simulink model "PE_main"  (R2025b)
settings: Solver=ode4  StartTime=0.0  StopTime=600  FixedStep=0.001  RelTol=1e-3
libraries: simulink x1
settings Model: Creator=manikantagonugondla  LastModifiedBy=manikantagonugondla

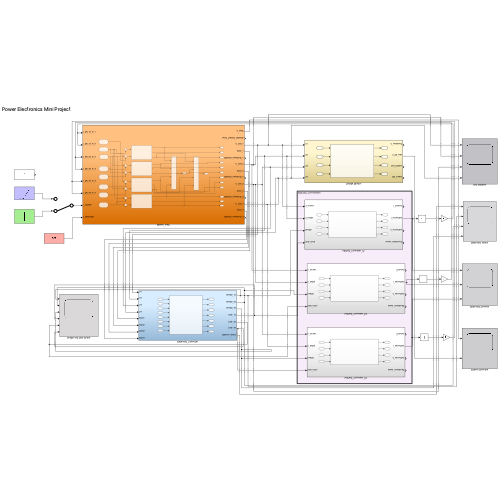
[thumbnail: Simulink's stored preview of the top-level diagram]
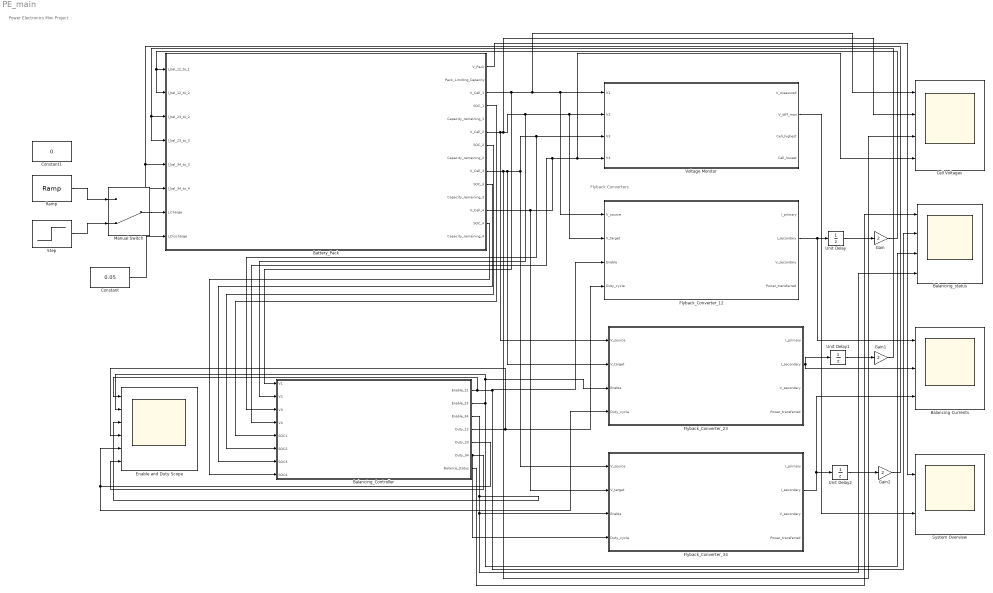
== system PE_main ==
  note: Power Electronics Mini Project
  note: Flyback Converters
  Balancing Currents : Scope  NumInputPorts=3
      settings: ActiveDisplayYMinimum=-7.6961589180783845  ActiveDisplayYMaximum=7.5868246502245036  DataLoggingVariableName=ScopeData2
  Balancing_Controller : Subsystem
  Balancing_status : Scope  NumInputPorts=4
      settings: ActiveDisplayYMinimum=1.1215595122943847  ActiveDisplayYMaximum=2.0976044986339573
  Battery_Pack : Subsystem
  Cell Voltages : Scope  NumInputPorts=4
      settings: ActiveDisplayYMinimum=2.624907670031094  ActiveDisplayYMaximum=4.321195310518152
  Constant : Constant  Value=0.05
  Constant1 : Constant  Value=0
  Enable and Duty Scope : Scope  NumInputPorts=6
      settings: ActiveDisplayYMinimum=-0.12499999999999997  ActiveDisplayYMaximum=1.125  DataLoggingVariableName=ScopeData4
  Flyback_Converter_12 : Subsystem
  Flyback_Converter_23 : Subsystem
  Flyback_Converter_34 : Subsystem
  Gain : Gain  Gain=2
  Gain1 : Gain  Gain=2
  Gain2 : Gain  Gain=2
  Manual Switch : ManualSwitch  CurrentSetting=0
  Ramp : simulink/Sources/Ramp  slope=0.01  start=100  InitialOutput=0
  Step : Step  Time=200  After=0.5  SampleTime=0
  System Overview : Scope  NumInputPorts=2
      settings: ActiveDisplayYMinimum=13.339480983921661  ActiveDisplayYMaximum=13.76875860674742  DataLoggingVariableName=ScopeData3
  Unit Delay : UnitDelay  SampleTime=-1  HasFrameUpgradeWarning=on
  Unit Delay1 : UnitDelay  SampleTime=-1  HasFrameUpgradeWarning=on
  Unit Delay2 : UnitDelay  SampleTime=-1  HasFrameUpgradeWarning=on
  Voltage Monitor : Subsystem
  wires:
  Battery_Pack/9(V_Cell_3) -> Cell Voltages/3, Flyback_Converter_23/2(V_target), Balancing_Controller/3(V3), Voltage Monitor/3(V3), Flyback_Converter_34/1(V_source)
  Battery_Pack/12(V_Cell_4) -> Flyback_Converter_34/2(V_target), Balancing_Controller/4(V4), Cell Voltages/4, Voltage Monitor/4(V4)
  Battery_Pack/4(SOC_1) -> Balancing_Controller/5(SOC1)
  Battery_Pack/7(SOC_2) -> Balancing_Controller/6(SOC2)
  Battery_Pack/10(SOC_3) -> Balancing_Controller/7(SOC3)
  Battery_Pack/13(SOC_4) -> Balancing_Controller/8(SOC4)
  Balancing_Controller/2(Enable_23) -> Enable and Duty Scope/2, Flyback_Converter_23/3(Enable), Balancing_status/3
  Balancing_Controller/3(Enable_34) -> Balancing_status/4, Flyback_Converter_34/3(Enable), Enable and Duty Scope/3
  Balancing_Controller/5(Duty_23) -> Enable and Duty Scope/5, Flyback_Converter_23/4(Duty_cycle)
  Balancing_Controller/6(Duty_34) -> Enable and Duty Scope/6, Flyback_Converter_34/4(Duty_cycle)
  Balancing_Controller/7(Balance_status) -> Balancing_status/1
  Flyback_Converter_12/2(I_secondary) -> Unit Delay/1, Balancing Currents/1
  Flyback_Converter_23/2(I_secondary) -> Unit Delay1/1, Balancing Currents/2
  Flyback_Converter_34/2(I_secondary) -> Balancing Currents/3, Unit Delay2/1
  Battery_Pack/1(V_Pack) -> System Overview/1
  Voltage Monitor/2(V_diff_max) -> System Overview/2
  Constant/1 -> Battery_Pack/8(I_Discharge)
  Gain/1 -> Battery_Pack/2(I_bal_12_to_2), Battery_Pack/1(I_bal_12_to_1)
  Gain2/1 -> Battery_Pack/6(I_bal_34_to_4), Battery_Pack/5(I_bal_34_to_3)
  Unit Delay/1 -> Gain/1
  Unit Delay1/1 -> Gain1/1
  Unit Delay2/1 -> Gain2/1
  Gain1/1 -> Battery_Pack/4(I_bal_23_to_3), Battery_Pack/3(I_bal_23_to_2)
  Battery_Pack/6(V_Cell_2) -> Flyback_Converter_23/1(V_source), Cell Voltages/2, Balancing_Controller/2(V2), Flyback_Converter_12/2(V_target), Voltage Monitor/2(V2)
  Battery_Pack/3(V_Cell_1) -> Balancing_Controller/1(V1), Cell Voltages/1, Flyback_Converter_12/1(V_source), Voltage Monitor/1(V1)
  Balancing_Controller/1(Enable_12) -> Enable and Duty Scope/1, Flyback_Converter_12/3(Enable), Balancing_status/2
  Balancing_Controller/4(Duty_12) -> Enable and Duty Scope/4, Flyback_Converter_12/4(Duty_cycle)
  Ramp/1 -> Manual Switch/1
  Step/1 -> Manual Switch/2
  Manual Switch/1 -> Battery_Pack/7(I_Charge)

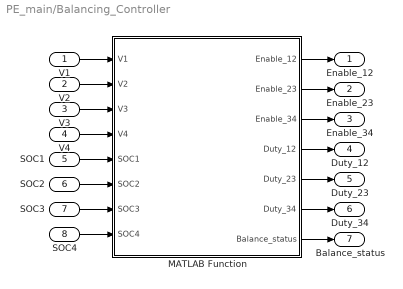
== system PE_main/Balancing_Controller ==
  V1 : Inport
  V2 : Inport  Port=2
  V3 : Inport  Port=3
  V4 : Inport  Port=4
  SOC1 : Inport  Port=5
  SOC2 : Inport  Port=6
  SOC3 : Inport  Port=7
  SOC4 : Inport  Port=8
  MATLAB Function : MATLAB Function  TreatAsAtomicUnit=on
  Enable_12 : Outport
  Enable_23 : Outport  Port=2
  Enable_34 : Outport  Port=3
  Duty_12 : Outport  Port=4
  Duty_23 : Outport  Port=5
  Duty_34 : Outport  Port=6
  Balance_status : Outport  Port=7
  wires:
  V1/1 -> MATLAB Function/1(V1)
  MATLAB Function/1(Enable_12) -> Enable_12/1
  V2/1 -> MATLAB Function/2(V2)
  V3/1 -> MATLAB Function/3(V3)
  V4/1 -> MATLAB Function/4(V4)
  SOC1/1 -> MATLAB Function/5(SOC1)
  SOC2/1 -> MATLAB Function/6(SOC2)
  SOC3/1 -> MATLAB Function/7(SOC3)
  SOC4/1 -> MATLAB Function/8(SOC4)
  MATLAB Function/2(Enable_23) -> Enable_23/1
  MATLAB Function/3(Enable_34) -> Enable_34/1
  MATLAB Function/4(Duty_12) -> Duty_12/1
  MATLAB Function/5(Duty_23) -> Duty_23/1
  MATLAB Function/6(Duty_34) -> Duty_34/1
  MATLAB Function/7(Balance_status) -> Balance_status/1

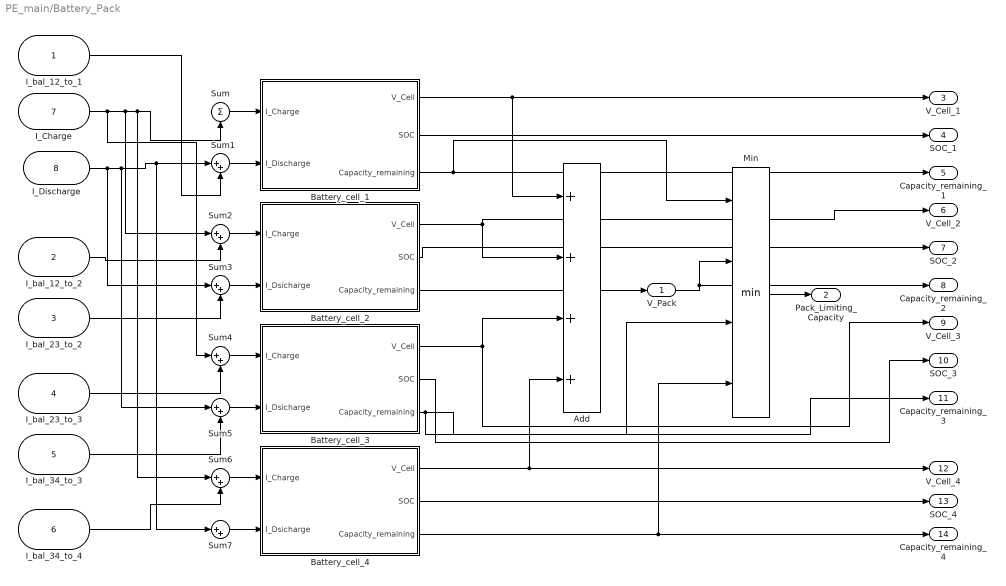
== system PE_main/Battery_Pack ==
  I_bal_12_to_1 : Inport
  I_bal_12_to_2 : Inport  Port=2
  I_bal_23_to_2 : Inport  Port=3
  I_bal_23_to_3 : Inport  Port=4
  I_bal_34_to_3 : Inport  Port=5
  I_bal_34_to_4 : Inport  Port=6
  I_Charge : Inport  Port=7
  I_Discharge : Inport  Port=8
  Add : Sum  Inputs=++++
  Battery_cell_1 : Subsystem
  Battery_cell_2 : Subsystem
  Battery_cell_3 : Subsystem
  Battery_cell_4 : Subsystem
  Min : MinMax  Inputs=4
  Sum : Sum  Inputs=|+
  Sum{1..7} (7 alike) : Sum  Inputs=|++
  V_Pack : Outport
  Pack_Limiting_Capacity : Outport  Port=2
  V_Cell_1 : Outport  Port=3
  SOC_1 : Outport  Port=4
  Capacity_remaining_1 : Outport  Port=5
  V_Cell_2 : Outport  Port=6
  SOC_2 : Outport  Port=7
  Capacity_remaining_2 : Outport  Port=8
  V_Cell_3 : Outport  Port=9
  SOC_3 : Outport  Port=10
  Capacity_remaining_3 : Outport  Port=11
  V_Cell_4 : Outport  Port=12
  SOC_4 : Outport  Port=13
  Capacity_remaining_4 : Outport  Port=14
  wires:
  Battery_cell_1/1(V_Cell) -> V_Cell_1/1, Add/1
  Battery_cell_2/1(V_Cell) -> Add/2, V_Cell_2/1
  Battery_cell_3/1(V_Cell) -> Add/3, V_Cell_3/1
  Battery_cell_4/1(V_Cell) -> V_Cell_4/1, Add/4
  Add/1 -> V_Pack/1
  Battery_cell_1/3(Capacity_remaining) -> Min/1, Capacity_remaining_1/1
  Battery_cell_2/3(Capacity_remaining) -> Min/2, Capacity_remaining_2/1
  Battery_cell_3/3(Capacity_remaining) -> Capacity_remaining_3/1, Min/3
  Battery_cell_4/3(Capacity_remaining) -> Capacity_remaining_4/1, Min/4
  Min/1 -> Pack_Limiting_Capacity/1
  Battery_cell_1/2(SOC) -> SOC_1/1
  Battery_cell_2/2(SOC) -> SOC_2/1
  Battery_cell_3/2(SOC) -> SOC_3/1
  Battery_cell_4/2(SOC) -> SOC_4/1
  I_Charge/1 -> Sum4/1, Sum2/1, Sum6/1, Sum/1
  Sum/1 -> Battery_cell_1/1(I_Charge)
  I_bal_12_to_1/1 -> Sum1/2
  I_Discharge/1 -> Sum5/1, Sum7/1, Sum1/1, Sum3/1
  Sum1/1 -> Battery_cell_1/2(I_Discharge)
  Sum2/1 -> Battery_cell_2/1(I_Charge)
  I_bal_12_to_2/1 -> Sum2/2
  I_bal_23_to_2/1 -> Sum3/2
  Sum3/1 -> Battery_cell_2/2(I_Dsicharge)
  I_bal_23_to_3/1 -> Sum4/2
  I_bal_34_to_3/1 -> Sum5/2
  I_bal_34_to_4/1 -> Sum6/2
  Sum4/1 -> Battery_cell_3/1(I_Charge)
  Sum5/1 -> Battery_cell_3/2(I_Dsicharge)
  Sum6/1 -> Battery_cell_4/1(I_Charge)
  Sum7/1 -> Battery_cell_4/2(I_Dsicharge)

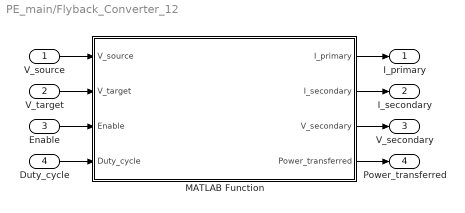
== system PE_main/Flyback_Converter_12 ==
  V_source : Inport
  V_target : Inport  Port=2
  Enable : Inport  Port=3
  Duty_cycle : Inport  Port=4
  MATLAB Function : MATLAB Function  TreatAsAtomicUnit=on
  I_primary : Outport
  I_secondary : Outport  Port=2
  V_secondary : Outport  Port=3
  Power_transferred : Outport  Port=4
  wires:
  V_source/1 -> MATLAB Function/1(V_source)
  MATLAB Function/1(I_primary) -> I_primary/1
  Enable/1 -> MATLAB Function/3(Enable)
  Duty_cycle/1 -> MATLAB Function/4(Duty_cycle)
  MATLAB Function/3(V_secondary) -> V_secondary/1
  MATLAB Function/2(I_secondary) -> I_secondary/1
  MATLAB Function/4(Power_transferred) -> Power_transferred/1
  V_target/1 -> MATLAB Function/2(V_target)

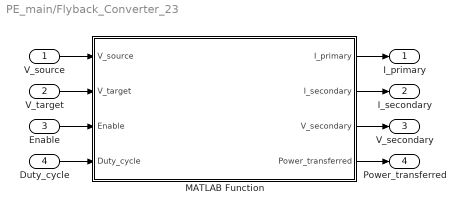
== system PE_main/Flyback_Converter_23 ==
  V_source : Inport
  V_target : Inport  Port=2
  Enable : Inport  Port=3
  Duty_cycle : Inport  Port=4
  MATLAB Function : MATLAB Function  TreatAsAtomicUnit=on
  I_primary : Outport
  I_secondary : Outport  Port=2
  V_secondary : Outport  Port=3
  Power_transferred : Outport  Port=4
  wires:
  V_source/1 -> MATLAB Function/1(V_source)
  MATLAB Function/1(I_primary) -> I_primary/1
  Enable/1 -> MATLAB Function/3(Enable)
  Duty_cycle/1 -> MATLAB Function/4(Duty_cycle)
  MATLAB Function/3(V_secondary) -> V_secondary/1
  MATLAB Function/2(I_secondary) -> I_secondary/1
  MATLAB Function/4(Power_transferred) -> Power_transferred/1
  V_target/1 -> MATLAB Function/2(V_target)

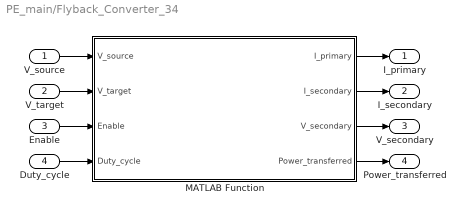
== system PE_main/Flyback_Converter_34 ==
  V_source : Inport
  V_target : Inport  Port=2
  Enable : Inport  Port=3
  Duty_cycle : Inport  Port=4
  MATLAB Function : MATLAB Function  TreatAsAtomicUnit=on
  I_primary : Outport
  I_secondary : Outport  Port=2
  V_secondary : Outport  Port=3
  Power_transferred : Outport  Port=4
  wires:
  V_source/1 -> MATLAB Function/1(V_source)
  MATLAB Function/1(I_primary) -> I_primary/1
  Enable/1 -> MATLAB Function/3(Enable)
  Duty_cycle/1 -> MATLAB Function/4(Duty_cycle)
  MATLAB Function/3(V_secondary) -> V_secondary/1
  MATLAB Function/2(I_secondary) -> I_secondary/1
  MATLAB Function/4(Power_transferred) -> Power_transferred/1
  V_target/1 -> MATLAB Function/2(V_target)

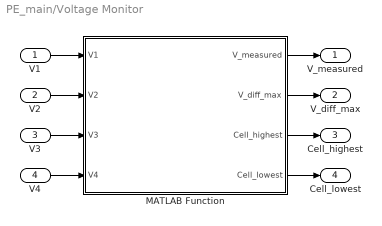
== system PE_main/Voltage Monitor ==
  V1 : Inport
  V2 : Inport  Port=2
  V3 : Inport  Port=3
  V4 : Inport  Port=4
  MATLAB Function : MATLAB Function  TreatAsAtomicUnit=on
  V_measured : Outport
  V_diff_max : Outport  Port=2
  Cell_highest : Outport  Port=3
  Cell_lowest : Outport  Port=4
  wires:
  V1/1 -> MATLAB Function/1(V1)
  V2/1 -> MATLAB Function/2(V2)
  V3/1 -> MATLAB Function/3(V3)
  V4/1 -> MATLAB Function/4(V4)
  MATLAB Function/2(V_diff_max) -> V_diff_max/1
  MATLAB Function/3(Cell_highest) -> Cell_highest/1
  MATLAB Function/1(V_measured) -> V_measured/1
  MATLAB Function/4(Cell_lowest) -> Cell_lowest/1

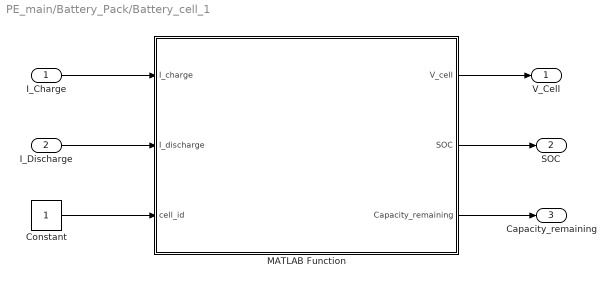
== system PE_main/Battery_Pack/Battery_cell_1 ==
  I_Charge : Inport
  I_Discharge : Inport  Port=2
  Constant : Constant
  MATLAB Function : MATLAB Function  TreatAsAtomicUnit=on
  V_Cell : Outport
  SOC : Outport  Port=2
  Capacity_remaining : Outport  Port=3
  wires:
  I_Discharge/1 -> MATLAB Function/2(I_discharge)
  I_Charge/1 -> MATLAB Function/1(I_charge)
  MATLAB Function/1(V_cell) -> V_Cell/1
  MATLAB Function/2(SOC) -> SOC/1
  MATLAB Function/3(Capacity_remaining) -> Capacity_remaining/1
  Constant/1 -> MATLAB Function/3(cell_id)

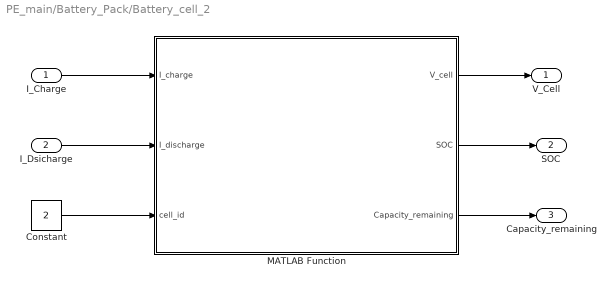
== system PE_main/Battery_Pack/Battery_cell_2 ==
  I_Charge : Inport
  I_Dsicharge : Inport  Port=2
  Constant : Constant  Value=2
  MATLAB Function : MATLAB Function  TreatAsAtomicUnit=on
  V_Cell : Outport
  SOC : Outport  Port=2
  Capacity_remaining : Outport  Port=3
  wires:
  I_Dsicharge/1 -> MATLAB Function/2(I_discharge)
  I_Charge/1 -> MATLAB Function/1(I_charge)
  MATLAB Function/1(V_cell) -> V_Cell/1
  MATLAB Function/2(SOC) -> SOC/1
  MATLAB Function/3(Capacity_remaining) -> Capacity_remaining/1
  Constant/1 -> MATLAB Function/3(cell_id)

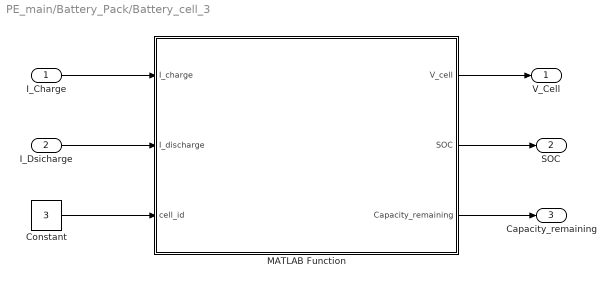
== system PE_main/Battery_Pack/Battery_cell_3 ==
  I_Charge : Inport
  I_Dsicharge : Inport  Port=2
  Constant : Constant  Value=3
  MATLAB Function : MATLAB Function  TreatAsAtomicUnit=on
  V_Cell : Outport
  SOC : Outport  Port=2
  Capacity_remaining : Outport  Port=3
  wires:
  I_Dsicharge/1 -> MATLAB Function/2(I_discharge)
  I_Charge/1 -> MATLAB Function/1(I_charge)
  MATLAB Function/1(V_cell) -> V_Cell/1
  MATLAB Function/2(SOC) -> SOC/1
  MATLAB Function/3(Capacity_remaining) -> Capacity_remaining/1
  Constant/1 -> MATLAB Function/3(cell_id)

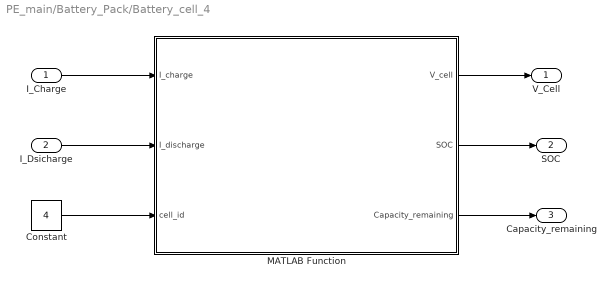
== system PE_main/Battery_Pack/Battery_cell_4 ==
  I_Charge : Inport
  I_Dsicharge : Inport  Port=2
  Constant : Constant  Value=4
  MATLAB Function : MATLAB Function  TreatAsAtomicUnit=on
  V_Cell : Outport
  SOC : Outport  Port=2
  Capacity_remaining : Outport  Port=3
  wires:
  I_Dsicharge/1 -> MATLAB Function/2(I_discharge)
  I_Charge/1 -> MATLAB Function/1(I_charge)
  MATLAB Function/1(V_cell) -> V_Cell/1
  MATLAB Function/2(SOC) -> SOC/1
  MATLAB Function/3(Capacity_remaining) -> Capacity_remaining/1
  Constant/1 -> MATLAB Function/3(cell_id)

== matlab function PE_main/Flyback_Converter_23/MATLAB Function ==
  data: V_source input; I_primary output; V_target input; Enable input; Duty_cycle input; I_secondary output; V_secondary output; Power_transferred output
function [I_primary, I_secondary, V_secondary, Power_transferred] = flyback_converter(V_source, V_target, Enable, Duty_cycle)
% Bidirectional Flyback Converter Model
% Automatically determines energy transfer direction based on voltage difference
% Energy flows from higher voltage cell to lower voltage cell

% Converter Parameters
L_primary = 100e-6;           % Primary inductance (100 µH)
N_ratio = 1.0;                % Turns ratio (1:1)
R_primary = 0.1;              % Primary winding resistance (Ohm)
R_secondary = 0.1;            % Secondary winding resistance (Ohm)
f_switching = 50e3;           % Switching frequency (50 kHz)
V_mosfet_drop = 0.1;          % MOSFET voltage drop (V)
V_diode_drop = 0.3;           % Diode voltage drop (V)
efficiency = 0.9;             % Energy transfer efficiency (90%)

% Persistent state variables
persistent I_L_state t_state;
if isempty(I_L_state)
    I_L_state = 0.0;
    t_state = 0.0;
end

% Time step and switching period
dt = 1e-5;                    % Fixed time step (10 µs)
t_state = t_state + dt;
T_switching = 1/f_switching;
t_normalized = mod(t_state, T_switching) / T_switching;

% Initialize outputs
I_primary = 0.0;
I_secondary = 0.0;
V_secondary = 0.0;
Power_transferred = 0.0;

% Determine energy transfer direction
V_diff = V_source - V_target;
voltage_threshold = 0.01;     % Minimum 10 mV difference to operate

% Check if converter should be active
converter_active = (Enable > 0.5) && (abs(V_diff) > voltage_threshold) && (Duty_cycle > 0.01);

if ~converter_active
    % Converter disabled - reset inductor current
    I_L_state = 0;
    return;
end

% Determine which cell is higher voltage (energy source)
if V_diff > 0
    % V_source > V_target: Forward direction
    % Energy flows from source to target
    V_high = V_source;
    V_low = V_target;
    direction = 1;  % Forward
else
    % V_target > V_source: Reverse direction
    % Energy flows from target to source
    V_high = V_target;
    V_low = V_source;
    direction = -1; % Reverse
end

% Generate switching signal
switch_on = (t_normalized < Duty_cycle);

if switch_on
    % ===== ENERGY STORAGE PHASE =====
    % MOSFET ON: Current builds up in primary inductance
    % Energy is stored in the magnetic field
    
    % Voltage across inductor (from high voltage cell)
    V_inductor = V_high - I_L_state * R_primary - V_mosfet_drop;
    
    % Rate of current change: V = L * di/dt
    dI_dt = V_inductor / L_primary;
    
    % Update inductor current
    I_L_state = max(0, I_L_state + dI_dt * dt);
    
    % Current flows through primary during this phase
    if direction > 0
        I_primary = I_L_state;
        I_secondary = 0;
    else
        I_primary = 0;
        I_secondary = -I_L_state; % Negative indicates reverse flow
    end
    
else
    % ===== ENERGY TRANSFER PHASE =====
    % MOSFET OFF: Stored energy transfers to secondary
    % Inductor current flows through secondary winding to low voltage cell
    
    if I_L_state > 0.01  % Only transfer if sufficient current exists
        
        % Calculate secondary current with transformer ratio and efficiency
        I_transferred = I_L_state * N_ratio * efficiency;
        
        % Voltage at secondary side
        V_secondary_actual = V_low + I_transferred * R_secondary + V_diode_drop;
        
        if direction > 0
            % Forward: Energy to target
            I_primary = 0;
            I_secondary = I_transferred;
            V_secondary = V_secondary_actual;
        else
            % Reverse: Energy to source
            I_primary = -I_transferred;
            I_secondary = 0;
            V_secondary = V_secondary_actual;
        end
        
        % Decay inductor current (energy has been transferred)
        % Exponential decay model
        decay_factor = 0.95;  % Faster decay for realistic behavior
        I_L_state = I_L_state * decay_factor;
        
    else
        % Current too low - reset
        I_L_state = 0;
    end
end

% Calculate instantaneous power transfer
if direction > 0
    Power_transferred = abs(I_secondary * V_target);
else
    Power_transferred = abs(I_primary * V_source);
end

end

== matlab function PE_main/Flyback_Converter_34/MATLAB Function ==
  data: V_source input; I_primary output; V_target input; Enable input; Duty_cycle input; I_secondary output; V_secondary output; Power_transferred output
function [I_primary, I_secondary, V_secondary, Power_transferred] = flyback_converter(V_source, V_target, Enable, Duty_cycle)
% Bidirectional Flyback Converter Model
% Automatically determines energy transfer direction based on voltage difference
% Energy flows from higher voltage cell to lower voltage cell

% Converter Parameters
L_primary = 100e-6;           % Primary inductance (100 µH)
N_ratio = 1.0;                % Turns ratio (1:1)
R_primary = 0.1;              % Primary winding resistance (Ohm)
R_secondary = 0.1;            % Secondary winding resistance (Ohm)
f_switching = 50e3;           % Switching frequency (50 kHz)
V_mosfet_drop = 0.1;          % MOSFET voltage drop (V)
V_diode_drop = 0.3;           % Diode voltage drop (V)
efficiency = 0.9;             % Energy transfer efficiency (90%)

% Persistent state variables
persistent I_L_state t_state;
if isempty(I_L_state)
    I_L_state = 0.0;
    t_state = 0.0;
end

% Time step and switching period
dt = 1e-5;                    % Fixed time step (10 µs)
t_state = t_state + dt;
T_switching = 1/f_switching;
t_normalized = mod(t_state, T_switching) / T_switching;

% Initialize outputs
I_primary = 0.0;
I_secondary = 0.0;
V_secondary = 0.0;
Power_transferred = 0.0;

% Determine energy transfer direction
V_diff = V_source - V_target;
voltage_threshold = 0.01;     % Minimum 10 mV difference to operate

% Check if converter should be active
converter_active = (Enable > 0.5) && (abs(V_diff) > voltage_threshold) && (Duty_cycle > 0.01);

if ~converter_active
    % Converter disabled - reset inductor current
    I_L_state = 0;
    return;
end

% Determine which cell is higher voltage (energy source)
if V_diff > 0
    % V_source > V_target: Forward direction
    % Energy flows from source to target
    V_high = V_source;
    V_low = V_target;
    direction = 1;  % Forward
else
    % V_target > V_source: Reverse direction
    % Energy flows from target to source
    V_high = V_target;
    V_low = V_source;
    direction = -1; % Reverse
end

% Generate switching signal
switch_on = (t_normalized < Duty_cycle);

if switch_on
    % ===== ENERGY STORAGE PHASE =====
    % MOSFET ON: Current builds up in primary inductance
    % Energy is stored in the magnetic field
    
    % Voltage across inductor (from high voltage cell)
    V_inductor = V_high - I_L_state * R_primary - V_mosfet_drop;
    
    % Rate of current change: V = L * di/dt
    dI_dt = V_inductor / L_primary;
    
    % Update inductor current
    I_L_state = max(0, I_L_state + dI_dt * dt);
    
    % Current flows through primary during this phase
    if direction > 0
        I_primary = I_L_state;
        I_secondary = 0;
    else
        I_primary = 0;
        I_secondary = -I_L_state; % Negative indicates reverse flow
    end
    
else
    % ===== ENERGY TRANSFER PHASE =====
    % MOSFET OFF: Stored energy transfers to secondary
    % Inductor current flows through secondary winding to low voltage cell
    
    if I_L_state > 0.01  % Only transfer if sufficient current exists
        
        % Calculate secondary current with transformer ratio and efficiency
        I_transferred = I_L_state * N_ratio * efficiency;
        
        % Voltage at secondary side
        V_secondary_actual = V_low + I_transferred * R_secondary + V_diode_drop;
        
        if direction > 0
            % Forward: Energy to target
            I_primary = 0;
            I_secondary = I_transferred;
            V_secondary = V_secondary_actual;
        else
            % Reverse: Energy to source
            I_primary = -I_transferred;
            I_secondary = 0;
            V_secondary = V_secondary_actual;
        end
        
        % Decay inductor current (energy has been transferred)
        % Exponential decay model
        decay_factor = 0.95;  % Faster decay for realistic behavior
        I_L_state = I_L_state * decay_factor;
        
    else
        % Current too low - reset
        I_L_state = 0;
    end
end

% Calculate instantaneous power transfer
if direction > 0
    Power_transferred = abs(I_secondary * V_target);
else
    Power_transferred = abs(I_primary * V_source);
end

end

== matlab function PE_main/Battery_Pack/Battery_cell_1/MATLAB Function ==
  data: I_charge input; V_cell output; I_discharge input; SOC output; Capacity_remaining output; cell_id input
function [V_cell, SOC, Capacity_remaining] = battery_cell_model(I_charge, I_discharge, cell_id)
%#codegen
% Lithium-ion Battery Cell Model
% Models voltage, SOC, and capacity with realistic variations

% Persistent state variables (retain values between function calls)
persistent SOC_state Capacity_Ah_state;

% Initialize persistent variables on first run
if isempty(SOC_state)
    % Set initial SOC based on cell ID to create imbalance
    if cell_id == 1
        SOC_state = 0.65;     % Cell 1: 65% SOC
    elseif cell_id == 2
        SOC_state = 0.70;     % Cell 2: 70% SOC (highest)
    elseif cell_id == 3
        SOC_state = 0.55;     % Cell 3: 55% SOC (lowest)
    else
        SOC_state = 0.60;     % Cell 4: 60% SOC
    end
end

if isempty(Capacity_Ah_state)
    % Cell capacities vary by ±5% (realistic manufacturing variation)
    base_capacity = 2.5;      % 2.5 Ah base capacity
    
    if cell_id == 1
        capacity_factor = 1.02;  % +2% (2.55 Ah)
    elseif cell_id == 2
        capacity_factor = 0.98;  % -2% (2.45 Ah)
    elseif cell_id == 3
        capacity_factor = 1.05;  % +5% (2.625 Ah)
    else
        capacity_factor = 0.97;  % -3% (2.425 Ah)
    end
    
    Capacity_Ah_state = base_capacity * capacity_factor;
end

% ===== BATTERY PARAMETERS =====
V_nominal = 3.7;              % Nominal voltage (V)
V_max = 4.2;                  % Maximum safe voltage (V)
V_min = 2.5;                  % Minimum safe voltage (V)
R_internal_base = 0.05;       % Base internal resistance (Ohm)
alpha = 0.3;                  % Resistance variation coefficient

% Internal resistance varies with SOC (increases as SOC decreases)
R_internal = R_internal_base * (1.0 + alpha * (1.0 - SOC_state));

% ===== NET CURRENT CALCULATION =====
% Positive I_net = charging, Negative I_net = discharging
I_net = I_charge - I_discharge;

% ===== SOC UPDATE =====
% Update SOC using current integration (Coulomb counting)
dt = 0.001;                   % Integration time step (1 ms)
dSOC = (I_net * dt) / (Capacity_Ah_state * 3600.0);  % Convert Ah to As
SOC_state = SOC_state + dSOC;

% Limit SOC to physical bounds [0, 1]
SOC_state = max(min(SOC_state, 1.0), 0.0);

% ===== OPEN CIRCUIT VOLTAGE CALCULATION =====
% Non-linear relationship between SOC and voltage
if SOC_state > 0.95
    % High SOC region (95-100%): voltage increases rapidly
    V_oc = V_max - 0.1 * (1.0 - SOC_state) / 0.05;
elseif SOC_state > 0.1
    % Normal operating region (10-95%): approximately linear
    V_oc = V_min + (V_nominal - V_min) * (SOC_state - 0.1) / 0.85 + 0.3 * SOC_state;
else
    % Low SOC region (0-10%): voltage drops rapidly
    V_oc = V_min + 0.2 * SOC_state / 0.1;
end

% ===== TERMINAL VOLTAGE =====
% Terminal voltage includes resistive voltage drop
V_cell = V_oc - I_net * R_internal;

% Ensure voltage stays within safe bounds
V_cell = max(min(V_cell, V_max), V_min);

% ===== OUTPUT CALCULATIONS =====
Capacity_remaining = SOC_state * Capacity_Ah_state;  % Remaining capacity (Ah)
SOC = SOC_state;                                      % Current SOC (0-1)

end

== matlab function PE_main/Voltage Monitor/MATLAB Function ==
  data: V1 input; V_measured output; V2 input; V3 input; V4 input; V_diff_max output; Cell_highest output; Cell_lowest output
function [V_measured, V_diff_max, Cell_highest, Cell_lowest] = voltage_monitor(V1, V2, V3, V4)
%#codegen

% Simulate real-world voltage measurement with noise and quantization
measurement_noise = 0.005;  % 5mV measurement noise (realistic for good ADCs)
ADC_resolution = 12;        % 12-bit ADC
V_ref = 5.0;               % ADC reference voltage

% Add measurement noise to simulate real sensors
V1_noisy = V1 + measurement_noise * (rand - 0.5);
V2_noisy = V2 + measurement_noise * (rand - 0.5);
V3_noisy = V3 + measurement_noise * (rand - 0.5);
V4_noisy = V4 + measurement_noise * (rand - 0.5);

% Simulate ADC quantization
ADC_step = V_ref / (2^ADC_resolution);
V1_quantized = round(V1_noisy / ADC_step) * ADC_step;
V2_quantized = round(V2_noisy / ADC_step) * ADC_step;
V3_quantized = round(V3_noisy / ADC_step) * ADC_step;
V4_quantized = round(V4_noisy / ADC_step) * ADC_step;

% Output measured voltages
V_measured = [V1_quantized, V2_quantized, V3_quantized, V4_quantized];

% Calculate voltage differences for balancing decisions
V_max = max(V_measured);
V_min = min(V_measured);
V_diff_max = V_max - V_min;

% Identify which cells need attention
[~, Cell_highest] = max(V_measured);
[~, Cell_lowest] = min(V_measured);

end

== matlab function PE_main/Battery_Pack/Battery_cell_2/MATLAB Function ==
  data: I_charge input; V_cell output; I_discharge input; SOC output; Capacity_remaining output; cell_id input
function [V_cell, SOC, Capacity_remaining] = battery_cell_model(I_charge, I_discharge, cell_id)
%#codegen
% Lithium-ion Battery Cell Model
% Models voltage, SOC, and capacity with realistic variations

% Persistent state variables (retain values between function calls)
persistent SOC_state Capacity_Ah_state;

% Initialize persistent variables on first run
if isempty(SOC_state)
    % Set initial SOC based on cell ID to create imbalance
    if cell_id == 1
        SOC_state = 0.65;     % Cell 1: 65% SOC
    elseif cell_id == 2
        SOC_state = 0.70;     % Cell 2: 70% SOC (highest)
    elseif cell_id == 3
        SOC_state = 0.55;     % Cell 3: 55% SOC (lowest)
    else
        SOC_state = 0.60;     % Cell 4: 60% SOC
    end
end

if isempty(Capacity_Ah_state)
    % Cell capacities vary by ±5% (realistic manufacturing variation)
    base_capacity = 2.5;      % 2.5 Ah base capacity
    
    if cell_id == 1
        capacity_factor = 1.02;  % +2% (2.55 Ah)
    elseif cell_id == 2
        capacity_factor = 0.98;  % -2% (2.45 Ah)
    elseif cell_id == 3
        capacity_factor = 1.05;  % +5% (2.625 Ah)
    else
        capacity_factor = 0.97;  % -3% (2.425 Ah)
    end
    
    Capacity_Ah_state = base_capacity * capacity_factor;
end

% ===== BATTERY PARAMETERS =====
V_nominal = 3.7;              % Nominal voltage (V)
V_max = 4.2;                  % Maximum safe voltage (V)
V_min = 2.5;                  % Minimum safe voltage (V)
R_internal_base = 0.05;       % Base internal resistance (Ohm)
alpha = 0.3;                  % Resistance variation coefficient

% Internal resistance varies with SOC (increases as SOC decreases)
R_internal = R_internal_base * (1.0 + alpha * (1.0 - SOC_state));

% ===== NET CURRENT CALCULATION =====
% Positive I_net = charging, Negative I_net = discharging
I_net = I_charge - I_discharge;

% ===== SOC UPDATE =====
% Update SOC using current integration (Coulomb counting)
dt = 0.001;                   % Integration time step (1 ms)
dSOC = (I_net * dt) / (Capacity_Ah_state * 3600.0);  % Convert Ah to As
SOC_state = SOC_state + dSOC;

% Limit SOC to physical bounds [0, 1]
SOC_state = max(min(SOC_state, 1.0), 0.0);

% ===== OPEN CIRCUIT VOLTAGE CALCULATION =====
% Non-linear relationship between SOC and voltage
if SOC_state > 0.95
    % High SOC region (95-100%): voltage increases rapidly
    V_oc = V_max - 0.1 * (1.0 - SOC_state) / 0.05;
elseif SOC_state > 0.1
    % Normal operating region (10-95%): approximately linear
    V_oc = V_min + (V_nominal - V_min) * (SOC_state - 0.1) / 0.85 + 0.3 * SOC_state;
else
    % Low SOC region (0-10%): voltage drops rapidly
    V_oc = V_min + 0.2 * SOC_state / 0.1;
end

% ===== TERMINAL VOLTAGE =====
% Terminal voltage includes resistive voltage drop
V_cell = V_oc - I_net * R_internal;

% Ensure voltage stays within safe bounds
V_cell = max(min(V_cell, V_max), V_min);

% ===== OUTPUT CALCULATIONS =====
Capacity_remaining = SOC_state * Capacity_Ah_state;  % Remaining capacity (Ah)
SOC = SOC_state;                                      % Current SOC (0-1)

end

== matlab function PE_main/Battery_Pack/Battery_cell_3/MATLAB Function ==
  data: I_charge input; V_cell output; I_discharge input; SOC output; Capacity_remaining output; cell_id input
function [V_cell, SOC, Capacity_remaining] = battery_cell_model(I_charge, I_discharge, cell_id)
%#codegen
% Lithium-ion Battery Cell Model
% Models voltage, SOC, and capacity with realistic variations

% Persistent state variables (retain values between function calls)
persistent SOC_state Capacity_Ah_state;

% Initialize persistent variables on first run
if isempty(SOC_state)
    % Set initial SOC based on cell ID to create imbalance
    if cell_id == 1
        SOC_state = 0.65;     % Cell 1: 65% SOC
    elseif cell_id == 2
        SOC_state = 0.70;     % Cell 2: 70% SOC (highest)
    elseif cell_id == 3
        SOC_state = 0.55;     % Cell 3: 55% SOC (lowest)
    else
        SOC_state = 0.60;     % Cell 4: 60% SOC
    end
end

if isempty(Capacity_Ah_state)
    % Cell capacities vary by ±5% (realistic manufacturing variation)
    base_capacity = 2.5;      % 2.5 Ah base capacity
    
    if cell_id == 1
        capacity_factor = 1.02;  % +2% (2.55 Ah)
    elseif cell_id == 2
        capacity_factor = 0.98;  % -2% (2.45 Ah)
    elseif cell_id == 3
        capacity_factor = 1.05;  % +5% (2.625 Ah)
    else
        capacity_factor = 0.97;  % -3% (2.425 Ah)
    end
    
    Capacity_Ah_state = base_capacity * capacity_factor;
end

% ===== BATTERY PARAMETERS =====
V_nominal = 3.7;              % Nominal voltage (V)
V_max = 4.2;                  % Maximum safe voltage (V)
V_min = 2.5;                  % Minimum safe voltage (V)
R_internal_base = 0.05;       % Base internal resistance (Ohm)
alpha = 0.3;                  % Resistance variation coefficient

% Internal resistance varies with SOC (increases as SOC decreases)
R_internal = R_internal_base * (1.0 + alpha * (1.0 - SOC_state));

% ===== NET CURRENT CALCULATION =====
% Positive I_net = charging, Negative I_net = discharging
I_net = I_charge - I_discharge;

% ===== SOC UPDATE =====
% Update SOC using current integration (Coulomb counting)
dt = 0.001;                   % Integration time step (1 ms)
dSOC = (I_net * dt) / (Capacity_Ah_state * 3600.0);  % Convert Ah to As
SOC_state = SOC_state + dSOC;

% Limit SOC to physical bounds [0, 1]
SOC_state = max(min(SOC_state, 1.0), 0.0);

% ===== OPEN CIRCUIT VOLTAGE CALCULATION =====
% Non-linear relationship between SOC and voltage
if SOC_state > 0.95
    % High SOC region (95-100%): voltage increases rapidly
    V_oc = V_max - 0.1 * (1.0 - SOC_state) / 0.05;
elseif SOC_state > 0.1
    % Normal operating region (10-95%): approximately linear
    V_oc = V_min + (V_nominal - V_min) * (SOC_state - 0.1) / 0.85 + 0.3 * SOC_state;
else
    % Low SOC region (0-10%): voltage drops rapidly
    V_oc = V_min + 0.2 * SOC_state / 0.1;
end

% ===== TERMINAL VOLTAGE =====
% Terminal voltage includes resistive voltage drop
V_cell = V_oc - I_net * R_internal;

% Ensure voltage stays within safe bounds
V_cell = max(min(V_cell, V_max), V_min);

% ===== OUTPUT CALCULATIONS =====
Capacity_remaining = SOC_state * Capacity_Ah_state;  % Remaining capacity (Ah)
SOC = SOC_state;                                      % Current SOC (0-1)

end

== matlab function PE_main/Battery_Pack/Battery_cell_4/MATLAB Function ==
  data: I_charge input; V_cell output; I_discharge input; SOC output; Capacity_remaining output; cell_id input
function [V_cell, SOC, Capacity_remaining] = battery_cell_model(I_charge, I_discharge, cell_id)
%#codegen
% Lithium-ion Battery Cell Model
% Models voltage, SOC, and capacity with realistic variations

% Persistent state variables (retain values between function calls)
persistent SOC_state Capacity_Ah_state;

% Initialize persistent variables on first run
if isempty(SOC_state)
    % Set initial SOC based on cell ID to create imbalance
    if cell_id == 1
        SOC_state = 0.65;     % Cell 1: 65% SOC
    elseif cell_id == 2
        SOC_state = 0.70;     % Cell 2: 70% SOC (highest)
    elseif cell_id == 3
        SOC_state = 0.55;     % Cell 3: 55% SOC (lowest)
    else
        SOC_state = 0.60;     % Cell 4: 60% SOC
    end
end

if isempty(Capacity_Ah_state)
    % Cell capacities vary by ±5% (realistic manufacturing variation)
    base_capacity = 2.5;      % 2.5 Ah base capacity
    
    if cell_id == 1
        capacity_factor = 1.02;  % +2% (2.55 Ah)
    elseif cell_id == 2
        capacity_factor = 0.98;  % -2% (2.45 Ah)
    elseif cell_id == 3
        capacity_factor = 1.05;  % +5% (2.625 Ah)
    else
        capacity_factor = 0.97;  % -3% (2.425 Ah)
    end
    
    Capacity_Ah_state = base_capacity * capacity_factor;
end

% ===== BATTERY PARAMETERS =====
V_nominal = 3.7;              % Nominal voltage (V)
V_max = 4.2;                  % Maximum safe voltage (V)
V_min = 2.5;                  % Minimum safe voltage (V)
R_internal_base = 0.05;       % Base internal resistance (Ohm)
alpha = 0.3;                  % Resistance variation coefficient

% Internal resistance varies with SOC (increases as SOC decreases)
R_internal = R_internal_base * (1.0 + alpha * (1.0 - SOC_state));

% ===== NET CURRENT CALCULATION =====
% Positive I_net = charging, Negative I_net = discharging
I_net = I_charge - I_discharge;

% ===== SOC UPDATE =====
% Update SOC using current integration (Coulomb counting)
dt = 0.001;                   % Integration time step (1 ms)
dSOC = (I_net * dt) / (Capacity_Ah_state * 3600.0);  % Convert Ah to As
SOC_state = SOC_state + dSOC;

% Limit SOC to physical bounds [0, 1]
SOC_state = max(min(SOC_state, 1.0), 0.0);

% ===== OPEN CIRCUIT VOLTAGE CALCULATION =====
% Non-linear relationship between SOC and voltage
if SOC_state > 0.95
    % High SOC region (95-100%): voltage increases rapidly
    V_oc = V_max - 0.1 * (1.0 - SOC_state) / 0.05;
elseif SOC_state > 0.1
    % Normal operating region (10-95%): approximately linear
    V_oc = V_min + (V_nominal - V_min) * (SOC_state - 0.1) / 0.85 + 0.3 * SOC_state;
else
    % Low SOC region (0-10%): voltage drops rapidly
    V_oc = V_min + 0.2 * SOC_state / 0.1;
end

% ===== TERMINAL VOLTAGE =====
% Terminal voltage includes resistive voltage drop
V_cell = V_oc - I_net * R_internal;

% Ensure voltage stays within safe bounds
V_cell = max(min(V_cell, V_max), V_min);

% ===== OUTPUT CALCULATIONS =====
Capacity_remaining = SOC_state * Capacity_Ah_state;  % Remaining capacity (Ah)
SOC = SOC_state;                                      % Current SOC (0-1)

end

== matlab function PE_main/Flyback_Converter_12/MATLAB Function ==
  data: V_source input; I_primary output; V_target input; Enable input; Duty_cycle input; I_secondary output; V_secondary output; Power_transferred output
function [I_primary, I_secondary, V_secondary, Power_transferred] = flyback_converter(V_source, V_target, Enable, Duty_cycle)
% Bidirectional Flyback Converter Model
% Automatically determines energy transfer direction based on voltage difference
% Energy flows from higher voltage cell to lower voltage cell

% Converter Parameters
L_primary = 100e-6;           % Primary inductance (100 µH)
N_ratio = 1.0;                % Turns ratio (1:1)
R_primary = 0.1;              % Primary winding resistance (Ohm)
R_secondary = 0.1;            % Secondary winding resistance (Ohm)
f_switching = 50e3;           % Switching frequency (50 kHz)
V_mosfet_drop = 0.1;          % MOSFET voltage drop (V)
V_diode_drop = 0.3;           % Diode voltage drop (V)
efficiency = 0.9;             % Energy transfer efficiency (90%)

% Persistent state variables
persistent I_L_state t_state;
if isempty(I_L_state)
    I_L_state = 0.0;
    t_state = 0.0;
end

% Time step and switching period
dt = 1e-5;                    % Fixed time step (10 µs)
t_state = t_state + dt;
T_switching = 1/f_switching;
t_normalized = mod(t_state, T_switching) / T_switching;

% Initialize outputs
I_primary = 0.0;
I_secondary = 0.0;
V_secondary = 0.0;
Power_transferred = 0.0;

% Determine energy transfer direction
V_diff = V_source - V_target;
voltage_threshold = 0.01;     % Minimum 10 mV difference to operate

% Check if converter should be active
converter_active = (Enable > 0.5) && (abs(V_diff) > voltage_threshold) && (Duty_cycle > 0.01);

if ~converter_active
    % Converter disabled - reset inductor current
    I_L_state = 0;
    return;
end

% Determine which cell is higher voltage (energy source)
if V_diff > 0
    % V_source > V_target: Forward direction
    % Energy flows from source to target
    V_high = V_source;
    V_low = V_target;
    direction = 1;  % Forward
else
    % V_target > V_source: Reverse direction
    % Energy flows from target to source
    V_high = V_target;
    V_low = V_source;
    direction = -1; % Reverse
end

% Generate switching signal
switch_on = (t_normalized < Duty_cycle);

if switch_on
    % ===== ENERGY STORAGE PHASE =====
    % MOSFET ON: Current builds up in primary inductance
    % Energy is stored in the magnetic field
    
    % Voltage across inductor (from high voltage cell)
    V_inductor = V_high - I_L_state * R_primary - V_mosfet_drop;
    
    % Rate of current change: V = L * di/dt
    dI_dt = V_inductor / L_primary;
    
    % Update inductor current
    I_L_state = max(0, I_L_state + dI_dt * dt);
    
    % Current flows through primary during this phase
    if direction > 0
        I_primary = I_L_state;
        I_secondary = 0;
    else
        I_primary = 0;
        I_secondary = -I_L_state; % Negative indicates reverse flow
    end
    
else
    % ===== ENERGY TRANSFER PHASE =====
    % MOSFET OFF: Stored energy transfers to secondary
    % Inductor current flows through secondary winding to low voltage cell
    
    if I_L_state > 0.01  % Only transfer if sufficient current exists
        
        % Calculate secondary current with transformer ratio and efficiency
        I_transferred = I_L_state * N_ratio * efficiency;
        
        % Voltage at secondary side
        V_secondary_actual = V_low + I_transferred * R_secondary + V_diode_drop;
        
        if direction > 0
            % Forward: Energy to target
            I_primary = 0;
            I_secondary = I_transferred;
            V_secondary = V_secondary_actual;
        else
            % Reverse: Energy to source
            I_primary = -I_transferred;
            I_secondary = 0;
            V_secondary = V_secondary_actual;
        end
        
        % Decay inductor current (energy has been transferred)
        % Exponential decay model
        decay_factor = 0.95;  % Faster decay for realistic behavior
        I_L_state = I_L_state * decay_factor;
        
    else
        % Current too low - reset
        I_L_state = 0;
    end
end

% Calculate instantaneous power transfer
if direction > 0
    Power_transferred = abs(I_secondary * V_target);
else
    Power_transferred = abs(I_primary * V_source);
end

end

== matlab function PE_main/Balancing_Controller/MATLAB Function ==
  data: V1 input; Enable_12 output; V2 input; V3 input; V4 input; SOC1 input; SOC2 input; SOC3 input; SOC4 input; Enable_23 output; Enable_34 output; Duty_12 output; Duty_23 output; Duty_34 output; Balance_status output
function [Enable_12, Enable_23, Enable_34, Duty_12, Duty_23, Duty_34, Balance_status] = balancing_controller(V1, V2, V3, V4, SOC1, SOC2, SOC3, SOC4)
%#codegen
% Enhanced Balancing Controller
% Uses both voltage AND SOC for intelligent balancing decisions

% ===== CONTROL PARAMETERS =====
V_diff_threshold = 0.010;     % 10 mV - activation threshold
V_diff_stop = 0.05;          % 5 mV - stop threshold
SOC_diff_threshold = 0.02;    % 2% SOC difference threshold
Max_duty = 0.3;               % Maximum duty cycle (30%)
Kp_voltage = 3.0;             % Proportional gain for voltage control
Kp_SOC = 1.5;                 % Proportional gain for SOC control

% Initialize outputs
Enable_12 = 0; Enable_23 = 0; Enable_34 = 0;
Duty_12 = 0; Duty_23 = 0; Duty_34 = 0;
Balance_status = 0;

% ===== SAFETY CHECKS =====
V_cells = [V1, V2, V3, V4];
SOC_cells = [SOC1, SOC2, SOC3, SOC4];

% Check voltage limits
if any(V_cells > 4.15) || any(V_cells < 2.8)
    Balance_status = 2;  % Error state
    return;
end

% Check SOC limits
if any(SOC_cells > 0.95) || any(SOC_cells < 0.05)
    Balance_status = 2;  % Error state
    return;
end

% ===== CALCULATE DIFFERENCES =====
% Voltage differences between adjacent cells
V_diff_12 = abs(V1 - V2);
V_diff_23 = abs(V2 - V3);
V_diff_34 = abs(V3 - V4);

% SOC differences between adjacent cells
SOC_diff_12 = abs(SOC1 - SOC2);
SOC_diff_23 = abs(SOC2 - SOC3);
SOC_diff_34 = abs(SOC3 - SOC4);

% Calculate max difference across entire pack
V_max = max(V_cells);
V_min = min(V_cells);
V_diff_total = V_max - V_min;

SOC_max = max(SOC_cells);
SOC_min = min(SOC_cells);
SOC_diff_total = SOC_max - SOC_min;

% ===== BALANCING LOGIC =====
% Continue balancing until tight convergence
% Use BOTH voltage and SOC criteria

if (V_diff_total > V_diff_stop) || (SOC_diff_total > 0.01)
    
    % ----- Converter 12 (Cell 1 to Cell 2) -----
    if (V_diff_12 > V_diff_threshold) || (SOC_diff_12 > SOC_diff_threshold)
        Enable_12 = 1;
        
        % Calculate duty cycle based on both voltage and SOC
        duty_from_voltage = V_diff_12 * Kp_voltage;
        duty_from_SOC = SOC_diff_12 * Kp_SOC;
        
        % Use the larger of the two for faster balancing
        Duty_12 = min(max(duty_from_voltage, duty_from_SOC), Max_duty);
        
        Balance_status = 1;
    end
    
    % ----- Converter 23 (Cell 2 to Cell 3) -----
    if (V_diff_23 > V_diff_threshold) || (SOC_diff_23 > SOC_diff_threshold)
        Enable_23 = 1;
        
        duty_from_voltage = V_diff_23 * Kp_voltage;
        duty_from_SOC = SOC_diff_23 * Kp_SOC;
        
        Duty_23 = min(max(duty_from_voltage, duty_from_SOC), Max_duty);
        
        Balance_status = 1;
    end
    
    % ----- Converter 34 (Cell 3 to Cell 4) -----
    if (V_diff_34 > V_diff_threshold) || (SOC_diff_34 > SOC_diff_threshold)
        Enable_34 = 1;
        
        duty_from_voltage = V_diff_34 * Kp_voltage;
        duty_from_SOC = SOC_diff_34 * Kp_SOC;
        
        Duty_34 = min(max(duty_from_voltage, duty_from_SOC), Max_duty);
        
        Balance_status = 1;
    end
    
    % ----- AGGRESSIVE MODE -----
    % If total difference is large but no individual pair exceeds threshold,
    % activate the converter with the largest combined difference
    if Balance_status == 0 && ((V_diff_total > 0.02) || (SOC_diff_total > 0.03))
        
        % Calculate combined metric (voltage + SOC)
        metric_12 = V_diff_12 * 2 + SOC_diff_12;
        metric_23 = V_diff_23 * 2 + SOC_diff_23;
        metric_34 = V_diff_34 * 2 + SOC_diff_34;
        
        [max_metric, idx] = max([metric_12, metric_23, metric_34]);
        
        switch idx
            case 1  % Activate converter 12
                Enable_12 = 1;
                Duty_12 = min(max_metric * 0.5, Max_duty);
            case 2  % Activate converter 23
                Enable_23 = 1;
                Duty_23 = min(max_metric * 0.5, Max_duty);
            case 3  % Activate converter 34
                Enable_34 = 1;
                Duty_34 = min(max_metric * 0.5, Max_duty);
        end
        
        Balance_status = 1;
    end
end

% Output total voltage difference for monitoring (scaled for visibility)
Balance_status = min(V_diff_total * 100, 2);

end
